simulink library "simp_vd_lib"  (R2022b)
settings: Solver=VariableStepAuto  StartTime=0.0  StopTime=10.0  RelTol=1e-3
settings Model: Creator=LinF  LastModifiedBy=LinF

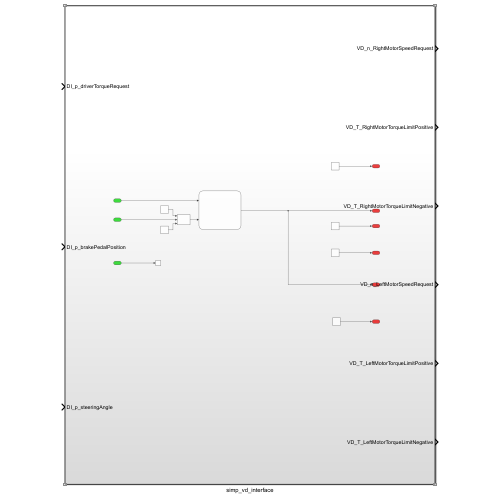
[thumbnail: Simulink's stored preview of the top-level diagram]
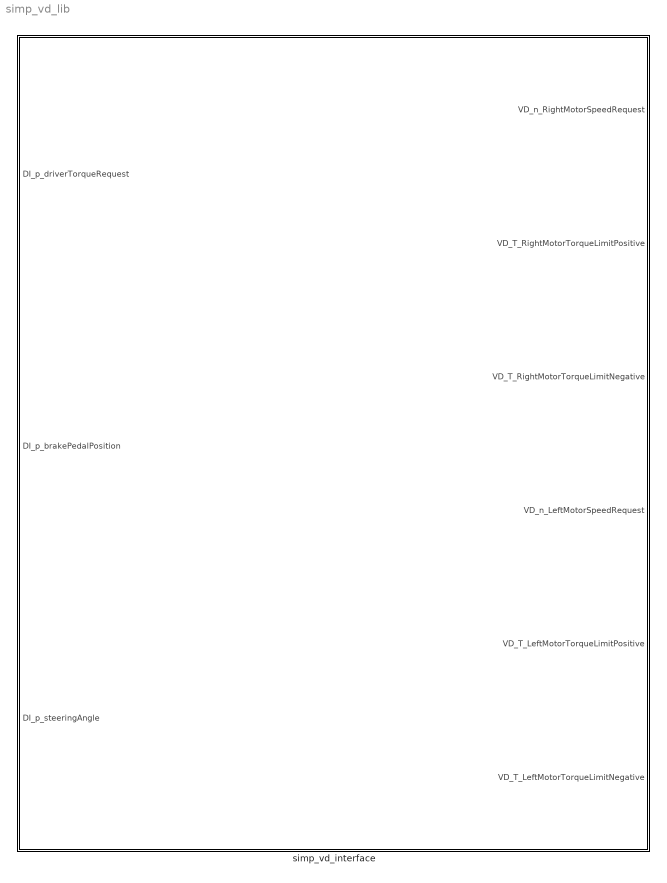
== system simp_vd_lib ==
  simp_vd_interface : Subsystem

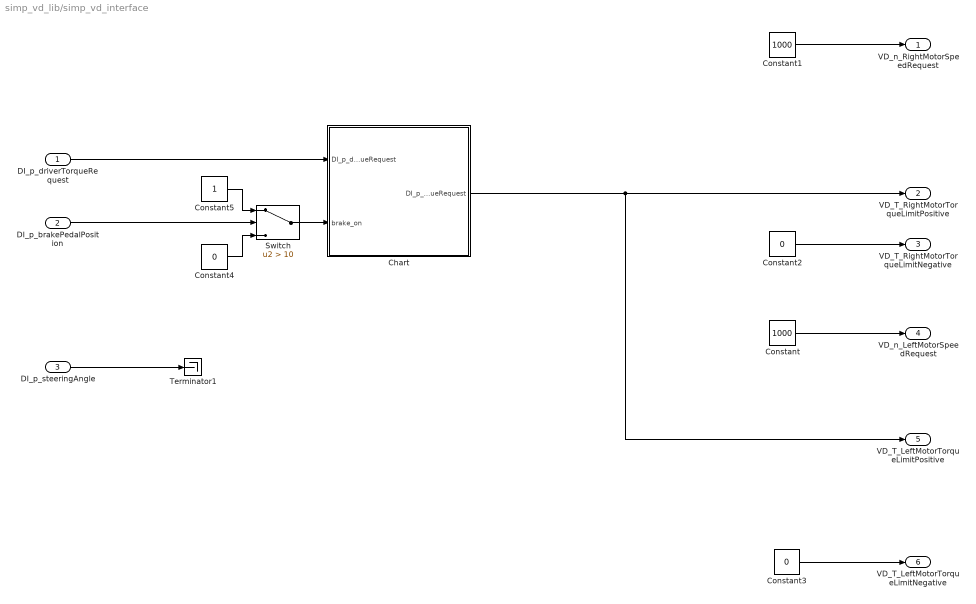
== system simp_vd_lib/simp_vd_interface ==
  DI_p_driverTorqueRequest : Inport
  DI_p_brakePedalPosition : Inport  Port=2
  DI_p_steeringAngle : Inport  Port=3
  Chart : Stateflow chart  TreatAsAtomicUnit=on
  Constant : Constant  Value=1000
  Constant1 : Constant  Value=1000
  Constant2 : Constant  Value=0
  Constant3 : Constant  Value=0
  Constant4 : Constant  Value=0
  Constant5 : Constant
  Switch : Switch  Criteria=u2 > Threshold  Threshold=10  SaturateOnIntegerOverflow=off  InputSameDT=off
  Terminator1 : Terminator
  VD_n_RightMotorSpeedRequest : Outport
  VD_T_RightMotorTorqueLimitPositive : Outport  Port=2
  VD_T_RightMotorTorqueLimitNegative : Outport  Port=3
  VD_n_LeftMotorSpeedRequest : Outport  Port=4
  VD_T_LeftMotorTorqueLimitPositive : Outport  Port=5
  VD_T_LeftMotorTorqueLimitNegative : Outport  Port=6
  wires:
  Chart/1(DI_p_motorTorqueRequest) -> VD_T_RightMotorTorqueLimitPositive/1, VD_T_LeftMotorTorqueLimitPositive/1
  DI_p_driverTorqueRequest/1 -> Chart/1(DI_p_driverTorqueRequest)
  DI_p_brakePedalPosition/1 -> Switch/2
  Switch/1 -> Chart/2(brake_on)
  Constant5/1 -> Switch/1
  Constant4/1 -> Switch/3
  Constant3/1 -> VD_T_LeftMotorTorqueLimitNegative/1
  Constant2/1 -> VD_T_RightMotorTorqueLimitNegative/1
  Constant1/1 -> VD_n_RightMotorSpeedRequest/1
  Constant/1 -> VD_n_LeftMotorSpeedRequest/1
  DI_p_steeringAngle/1 -> Terminator1/1

== stateflow chart simp_vd_lib/simp_vd_interface/Chart ==
  state Run
    en, du:
    DI_p_motorTorqueRequest = DI_p_driverTorqueRequest;
  state Stop
    en, du:
    DI_p_motorTorqueRequest = 0;
  (default) -> Run
  Run -> Stop : [DI_p_driverTorqueRequest >= 20 && brake_on]
  Stop -> Run : [DI_p_driverTorqueRequest < 5 && ~brake_on]
  data: DI_p_driverTorqueRequest input; brake_on input; DI_p_motorTorqueRequest output
